simulink library "courseFollow_cl"  (R2018b)
settings: Solver=VariableStepAuto  StartTime=0.0  StopTime=10.0  RelTol=1e-3
undefined symbols (not defined in the file): a
libraries: $bdroot x6, schmehlTangentRotation_ul x2, dspindex x1, vectorNormalizer_ul x1, angleBtw2DVecs_ul x1, tangVecToPath x1
settings Model: Creator=James Reed  LastModifiedBy=James Reed

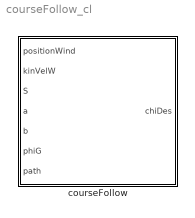
== system courseFollow_cl ==
  courseFollow : Subsystem

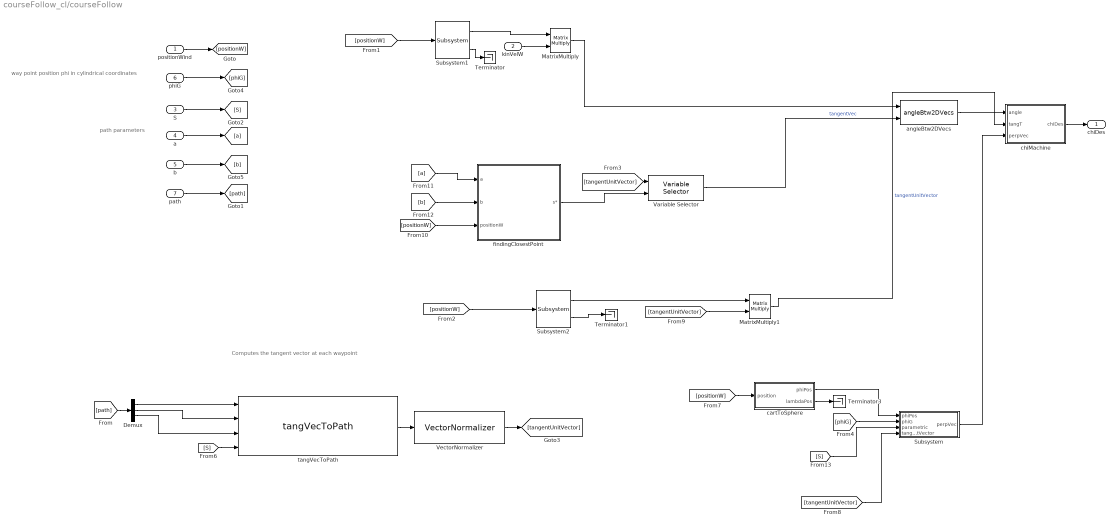
== system courseFollow_cl/courseFollow ==
  note: way point position phi in cylindrical coordinates
  note: path parameters
  note: Computes the tangent vector at each waypoint
  "positionWind " : Inport
  kinVelW : Inport  Port=2
  S : Inport  Port=3
  a : Inport  Port=4
  "b " : Inport  Port=5
  phiG : Inport  Port=6
  path : Inport  Port=7
  Demux : Demux  Outputs=3
  MatrixMultiply : Product  Multiplication=Matrix(*)
  MatrixMultiply1 : Product  Multiplication=Matrix(*)
  Subsystem : Subsystem
  Subsystem1 : schmehlTangentRotation_ul/Subsystem  SystemSampleTime=-1
  Subsystem2 : schmehlTangentRotation_ul/Subsystem  SystemSampleTime=-1
  Terminator : Terminator
  Terminator1 : Terminator
  Terminator3 : Terminator
  Variable Selector : dspindex/Variable Selector  NumInputs=1  rowsOrCols=Columns  IdxMode=Variable  Elements=[1 3]  ZerOneIdxMode=One-based  errmode=Clip Index  FillMode=on  FillValues=0
  "VectorNormalizer " : vectorNormalizer_ul/VectorNormalizer   SystemSampleTime=-1
  angleBtw2DVecs : angleBtw2DVecs_ul/angleBtw2DVecs  SystemSampleTime=-1
  cartToSphere : Subsystem
  chiMachine : Subsystem
  findingClosestPoint : Subsystem
  tangVecToPath : tangVecToPath/tangVecToPath  SystemSampleTime=-1
  "chiDes " : Outport
  wires:
  tangVecToPath/1 -> "VectorNormalizer "/1
  MatrixMultiply1/1 -> chiMachine/2(tangT)  "tangentUnitVector"
  Variable Selector/1 -> angleBtw2DVecs/2  "tangentVec"
  Subsystem1/2 -> Terminator/1
  kinVelW/1 -> MatrixMultiply/2
  Subsystem1/1 -> MatrixMultiply/1
  MatrixMultiply/1 -> angleBtw2DVecs/1
  Subsystem2/2 -> Terminator1/1
  "positionWind "/1 -> [positionW]
  [positionW] -> Subsystem1/1
  Subsystem2/1 -> MatrixMultiply1/1
  Demux/2 -> tangVecToPath/2
  Demux/3 -> tangVecToPath/3
  angleBtw2DVecs/1 -> chiMachine/1("angle ")
  chiMachine/1("chiDes ") -> "chiDes "/1
  cartToSphere/1(phiPos) -> Subsystem/1(phiPos)
  S/1 -> [S]
  [S] -> tangVecToPath/4
  [positionW] -> cartToSphere/1("position ")
  cartToSphere/2(lambdaPos) -> Terminator3/1
  "VectorNormalizer "/1 -> [tangentUnitVector]
  [tangentUnitVector] -> Subsystem/4("tangentUnitVector ")
  [tangentUnitVector] -> MatrixMultiply1/2
  [positionW] -> Subsystem2/1
  [positionW] -> findingClosestPoint/3(positionW)
  a/1 -> [a]
  "b "/1 -> [b]
  [a] -> findingClosestPoint/1(a)
  [b] -> findingClosestPoint/2(b)
  [S] -> Subsystem/3("parametric ")
  path/1 -> [path]
  [path] -> Demux/1
  Demux/1 -> tangVecToPath/1
  [tangentUnitVector] -> Variable Selector/1
  findingClosestPoint/1(s*) -> Variable Selector/2
  phiG/1 -> [phiG]
  Subsystem/1(perpVec) -> chiMachine/3("perpVec ")
  [phiG] -> Subsystem/2(phiG)

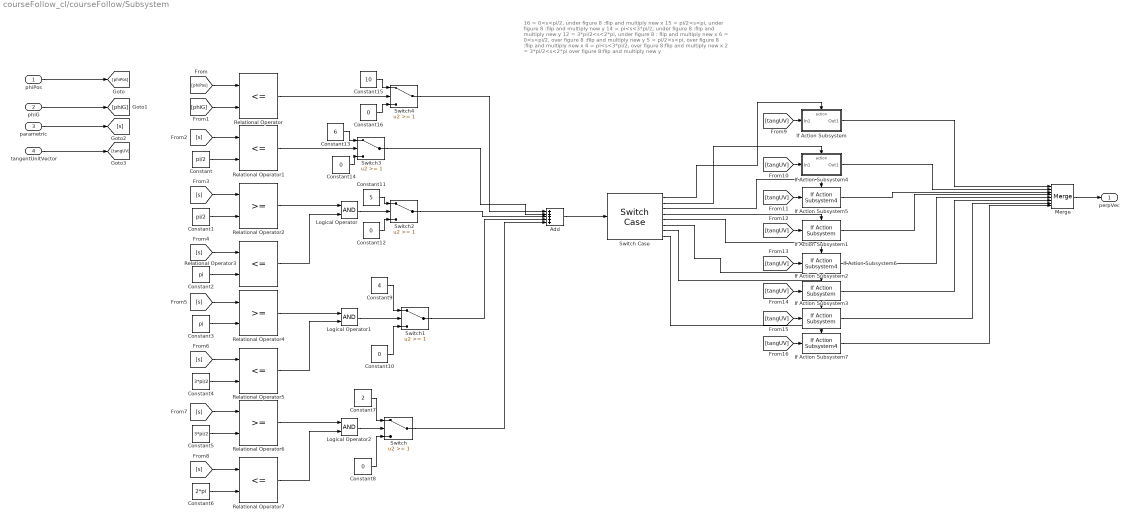
== system courseFollow_cl/courseFollow/Subsystem ==
  note: 16 = 0<s<pi/2, under figure 8 :flip and multiply new x
      | 15 = pi/2<s<pi, under figure 8  :flip and multiply new y
      | 14 = pi<s<3*pi/2, under figure 8 :flip and multiply new y
      | 12 = 3*pi/2<s<2*pi, under figure 8 : flip and multiply new x
      | 6 = 0<s<pi/2, over figure 8 :flip and multiply new y
      | 5 = pi/2<s<pi, over figure 8 :flip and multiply new x
      | 4 = pi<s<3*pi/2, over figure 8:flip and multiply new x
      | 2 = 3*pi/2<s<2*pi over figure 8:flip and multiply new y
  phiPos : Inport
  phiG : Inport  Port=2
  "parametric " : Inport  Port=3
  "tangentUnitVector " : Inport  Port=4
  Add : Sum  Inputs=+++++
  Constant : Constant  Value=pi/2
  Constant1 : Constant  Value=pi/2
  Constant{8,10,12,14,16} (5 alike) : Constant  Value=0
  Constant11 : Constant  Value=5
  Constant13 : Constant  Value=6
  Constant15 : Constant  Value=10
  Constant2 : Constant  Value=pi
  Constant3 : Constant  Value=pi
  Constant4 : Constant  Value=3*pi/2
  Constant5 : Constant  Value=3*pi/2
  Constant6 : Constant  Value=2*pi
  Constant7 : Constant  Value=2
  Constant9 : Constant  Value=4
  If Action Subsystem : Subsystem  TreatAsAtomicUnit=on
  If Action Subsystem1 : $bdroot/courseFollow/Subsystem/If Action Subsystem  SystemSampleTime=-1
  If Action Subsystem2 : $bdroot/courseFollow/Subsystem/If Action Subsystem  SystemSampleTime=-1
  If Action Subsystem3 : $bdroot/courseFollow/Subsystem/If Action Subsystem  SystemSampleTime=-1
  If Action Subsystem4 : Subsystem  TreatAsAtomicUnit=on
  If Action Subsystem5 : $bdroot/courseFollow/Subsystem/If Action Subsystem4  SystemSampleTime=-1
  If Action Subsystem6 : $bdroot/courseFollow/Subsystem/If Action Subsystem4  SystemSampleTime=-1
  If Action Subsystem7 : $bdroot/courseFollow/Subsystem/If Action Subsystem4  SystemSampleTime=-1
  Logical Operator : Logic  AllPortsSameDT=off  OutDataTypeStr=boolean
  Logical Operator1 : Logic  AllPortsSameDT=off  OutDataTypeStr=boolean
  Logical Operator2 : Logic  AllPortsSameDT=off  OutDataTypeStr=boolean
  Merge : Merge  Inputs=8
  Relational Operator{,1,3,5,7} (5 alike) : RelationalOperator  Operator=<=  OutDataTypeStr=boolean  RndMeth=Simplest
  Relational Operator2 : RelationalOperator  OutDataTypeStr=boolean  RndMeth=Simplest
  Relational Operator4 : RelationalOperator  OutDataTypeStr=boolean  RndMeth=Simplest
  Relational Operator6 : RelationalOperator  OutDataTypeStr=boolean  RndMeth=Simplest
  Switch{,1..4} (5 alike) : Switch  Threshold=1
  Switch Case : SwitchCase  CaseConditions={16,15,14,12,6,5,4,2}  ShowDefaultCase=off
  perpVec : Outport
  wires:
  phiPos/1 -> [phiPos]
  phiG/1 -> [phiG]
  Relational Operator/1 -> Switch4/2
  [phiPos] -> Relational Operator/1
  [phiG] -> Relational Operator/2
  "parametric "/1 -> [s]
  [s] -> Relational Operator1/1
  Constant/1 -> Relational Operator1/2
  [s] -> Relational Operator2/1
  Constant1/1 -> Relational Operator2/2
  Relational Operator2/1 -> Logical Operator/1
  [s] -> Relational Operator3/1
  Constant2/1 -> Relational Operator3/2
  Relational Operator3/1 -> Logical Operator/2
  Relational Operator4/1 -> Logical Operator1/1
  [s] -> Relational Operator4/1
  Constant4/1 -> Relational Operator5/2
  Constant3/1 -> Relational Operator4/2
  [s] -> Relational Operator5/1
  Relational Operator5/1 -> Logical Operator1/2
  Relational Operator6/1 -> Logical Operator2/1
  [s] -> Relational Operator6/1
  Constant6/1 -> Relational Operator7/2
  Constant5/1 -> Relational Operator6/2
  [s] -> Relational Operator7/1
  Relational Operator7/1 -> Logical Operator2/2
  Logical Operator2/1 -> Switch/2
  Constant7/1 -> Switch/1
  Constant8/1 -> Switch/3
  Logical Operator1/1 -> Switch1/2
  Constant9/1 -> Switch1/1
  Constant10/1 -> Switch1/3
  Logical Operator/1 -> Switch2/2
  Constant11/1 -> Switch2/1
  Constant12/1 -> Switch2/3
  Constant13/1 -> Switch3/1
  Constant14/1 -> Switch3/3
  Relational Operator1/1 -> Switch3/2
  Constant15/1 -> Switch4/1
  Constant16/1 -> Switch4/3
  Switch4/1 -> Add/1
  Switch3/1 -> Add/2
  Switch2/1 -> Add/3
  Switch1/1 -> Add/4
  Switch/1 -> Add/5
  Add/1 -> Switch Case/1
  Switch Case/1 -> If Action Subsystem/Action
  Switch Case/2 -> If Action Subsystem4/Action
  Switch Case/3 -> If Action Subsystem5/Action
  Switch Case/4 -> If Action Subsystem1/Action
  Switch Case/5 -> If Action Subsystem6/Action
  Switch Case/6 -> If Action Subsystem2/Action
  Switch Case/7 -> If Action Subsystem3/Action
  Switch Case/8 -> If Action Subsystem7/Action
  "tangentUnitVector "/1 -> [tangUV]
  [tangUV] -> If Action Subsystem/1(In1)
  [tangUV] -> If Action Subsystem4/1(In1)
  [tangUV] -> If Action Subsystem5/1
  [tangUV] -> If Action Subsystem1/1
  [tangUV] -> If Action Subsystem6/1
  [tangUV] -> If Action Subsystem2/1
  [tangUV] -> If Action Subsystem3/1
  [tangUV] -> If Action Subsystem7/1
  If Action Subsystem/1(Out1) -> Merge/1
  If Action Subsystem4/1(Out1) -> Merge/2
  If Action Subsystem5/1 -> Merge/3
  If Action Subsystem1/1 -> Merge/4
  If Action Subsystem6/1 -> Merge/5
  If Action Subsystem2/1 -> Merge/6
  If Action Subsystem3/1 -> Merge/7
  If Action Subsystem7/1 -> Merge/8
  Merge/1 -> perpVec/1

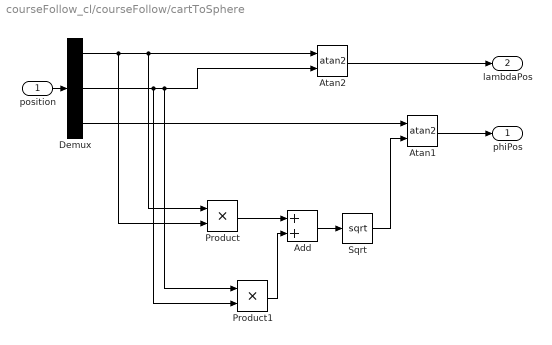
== system courseFollow_cl/courseFollow/cartToSphere ==
  "position " : Inport
  Add : Sum
  Atan1 : Trigonometry  Operator=atan2
  Atan2 : Trigonometry  Operator=atan2
  Demux : Demux  Outputs=3
  Product : Product
  Product1 : Product
  Sqrt : Sqrt  SaturateOnIntegerOverflow=on
  phiPos : Outport
  lambdaPos : Outport  Port=2
  wires:
  "position "/1 -> Demux/1
  Demux/1 -> Product/2, Product/1, Atan2/1
  Atan2/1 -> lambdaPos/1
  Demux/3 -> Atan1/1
  Atan1/1 -> phiPos/1
  Product/1 -> Add/1
  Add/1 -> Sqrt/1
  Demux/2 -> Product1/2, Product1/1, Atan2/2
  Product1/1 -> Add/2
  Sqrt/1 -> Atan1/2

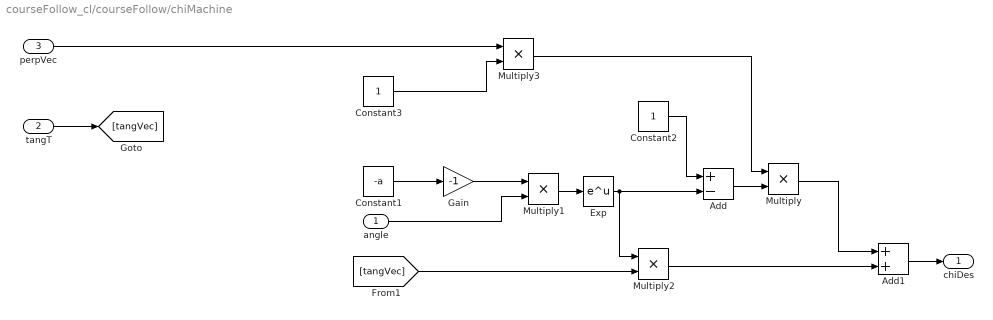
== system courseFollow_cl/courseFollow/chiMachine ==
  "angle " : Inport
  tangT : Inport  Port=2
  "perpVec " : Inport  Port=3
  Add : Sum  Inputs=+-
  Add1 : Sum
  Constant1 : Constant  Value=-a
  Constant2 : Constant
  Constant3 : Constant
  Exp : Math  SaturateOnIntegerOverflow=on
  Gain : Gain  Gain=-1
  Multiply{,1..3} (4 alike) : Product
  "chiDes " : Outport
  wires:
  tangT/1 -> [tangVec]
  Constant1/1 -> Gain/1
  Gain/1 -> Multiply1/1
  "angle "/1 -> Multiply1/2
  Multiply1/1 -> Exp/1
  Exp/1 -> Add/2, Multiply2/1
  Constant2/1 -> Add/1
  [tangVec] -> Multiply2/2
  Multiply3/1 -> Multiply/1
  Constant3/1 -> Multiply3/2
  Add/1 -> Multiply/2
  Multiply/1 -> Add1/1
  Multiply2/1 -> Add1/2
  Add1/1 -> "chiDes "/1
  "perpVec "/1 -> Multiply3/1

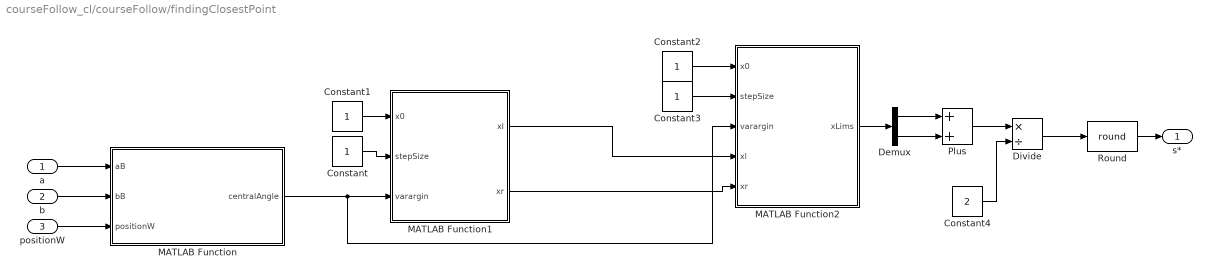
== system courseFollow_cl/courseFollow/findingClosestPoint ==
  a : Inport
  b : Inport  Port=2
  positionW : Inport  Port=3
  Constant{,1..3} (4 alike) : Constant
  Constant4 : Constant  Value=2
  Demux : Demux  Outputs=2
  Divide : Product  Inputs=*/
  MATLAB Function : MATLAB Function  TreatAsAtomicUnit=on
  MATLAB Function1 : MATLAB Function  TreatAsAtomicUnit=on
  MATLAB Function2 : MATLAB Function  TreatAsAtomicUnit=on
  Plus : Sum
  Round : Rounding  Operator=round
  s* : Outport
  wires:
  Constant2/1 -> MATLAB Function2/1(x0)
  Constant3/1 -> MATLAB Function2/2(stepSize)
  Constant1/1 -> MATLAB Function1/1(x0)
  Constant/1 -> MATLAB Function1/2(stepSize)
  MATLAB Function/1(centralAngle) -> MATLAB Function2/3(varargin), MATLAB Function1/3(varargin)
  MATLAB Function1/1(xl) -> MATLAB Function2/4(xl)
  MATLAB Function1/2(xr) -> MATLAB Function2/5(xr)
  MATLAB Function2/1(xLims) -> Demux/1
  Demux/2 -> Plus/2
  Demux/1 -> Plus/1
  Plus/1 -> Divide/1
  Constant4/1 -> Divide/2
  Divide/1 -> Round/1
  Round/1 -> s*/1
  a/1 -> MATLAB Function/1(aB)
  b/1 -> MATLAB Function/2(bB)
  positionW/1 -> MATLAB Function/3(positionW)

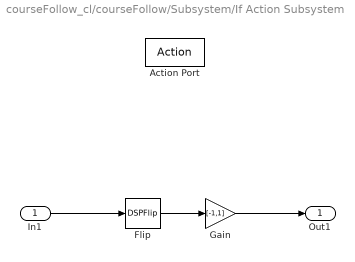
== system courseFollow_cl/courseFollow/Subsystem/If Action Subsystem ==
  In1 : Inport
  Action Port : ActionPort  ActionType=case
  Flip : DSPFlip
  Gain : Gain  Gain=[-1,1]
  Out1 : Outport
  wires:
  In1/1 -> Flip/1
  Flip/1 -> Gain/1
  Gain/1 -> Out1/1

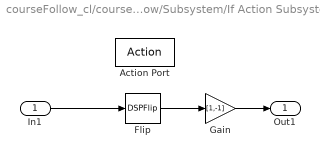
== system courseFollow_cl/courseFollow/Subsystem/If Action Subsystem4 ==
  In1 : Inport
  Action Port : ActionPort  ActionType=case
  Flip : DSPFlip
  Gain : Gain  Gain=[1,-1]
  Out1 : Outport
  wires:
  Flip/1 -> Gain/1
  In1/1 -> Flip/1
  Gain/1 -> Out1/1

== matlab function courseFollow_cl/courseFollow/findingClosestPoint/MATLAB Function ==
  data: aB input; centralAngle output; bB input; positionW input
function centralAngle  = fcn(aB,bB,positionW)

lambda_g = (aB.*sin(s))./(1 + ((aB/bB)^2).*(cos(s).^2)); %path longitude
phi_g  = (10*pi/180)+(((aB/bB)^2).*sin(s).*cos(s))./(1 + ((aB/bB)^2).*(cos(s).^2)); %path latitude

path = [ cos(lambda_g).*cos(phi_g);
         sin(lambda_g).*cos(phi_g);
         sin(phi_g);]; 
      pathFunction = @(s) path ;
     centralAngle = @(s)2*asin(.5*(norm(pathFunction(s)-currentPosition)));

== matlab function courseFollow_cl/courseFollow/findingClosestPoint/MATLAB Function1 ==
  data: x0 input; xl output; stepSize input; varargin input; xr output
function [xl,xr] = bound(x0, stepSize,varargin)

p = inputParser;

% Number of iterations before stopping attempt to tune step size
addOptional(p,'StepTimeout',1000,@(x) isnumeric(x) && isscalar(x))
% How much to increase the step size at every iteration
addOptional(p,'StepSizeMultiplier',2,@(x) isnumeric(x) && isscalar(x)  && x>=1)
% Number of iterations before quitting bounding phase
addOptional(p,'BoundingTimeout',1000,@(x) isnumeric(x) && isscalar(x))
% Handle of the function that you want to minimize
addOptional(p,'FunctionHandle',@objF,@(x) isa(x,'function_handle'))
% Initial point/guess
addRequired(p,'x0',@(x) isnumeric(x) && isvector(x))
% Step size
addRequired(p,'StepSize',@(x) isnumeric(x) && isscalar(x) && x>0)

parse(p,x0,stepSize,varargin{:})

fHandle  = p.Results.FunctionHandle;
stepSize = p.Results.StepSize;
x0       = p.Results.x0;

for tryCount = 1:p.Results.StepTimeout
    if fHandle(x0-stepSize) >= fHandle(x0) &&...
            fHandle(x0) >= fHandle(x0+stepSize)
        sign = +1;
        break
    elseif  fHandle(x0-stepSize) <= fHandle(x0) &&...
            fHandle(x0) <= fHandle(x0+stepSize)
        sign = -1;
        break
    end
    stepSize = stepSize/2^tryCount;
end

xCurrent = x0;
for ii = 0:p.Results.BoundingTimeout-1
    xRight = xCurrent + sign*stepSize*p.Results.StepSizeMultiplier^ii;
    if fHandle(xRight)>fHandle(xCurrent)
        break
    end
    xLeft = xCurrent;
    xCurrent = xRight;
end

if sign == -1
   xTemp  = sort([xLeft xRight]) ;
   xl  = xTemp(1);
   xr = xTemp(2);
end

end

== matlab function courseFollow_cl/courseFollow/findingClosestPoint/MATLAB Function2 ==
  data: x0 input; xLims output; stepSize input; varargin input; xl input; xr input
function xLims = goldenSection(x0,stepSize,varargin,xl,xr)
% Function to implement golden section to minimize a scalar function
%
% Required Inputs
% x0       - initial guess
% stepSize - initial step size (step size may be reduced if this is too
% big)
%
% Optional Inputs
% DisplayOutput -  true/false prints output to command window
% MaxIterations - Maximum number of iterations before quitting, default =
% 1000
% FunctionConvergence - convergence criteria for function value, set to
% zero to disable, default = 0.01
% InputConvergence - convergence criteria for function input, set to zero
% to disable, default = 0.01
% StepTimeout - Max number of iterations for bounding phase step size
% reduction, default = 1000
% BoundingTimeout - Max number of iterations for bounding phase, default =
% 1000
 

% Input parsing
p = inputParser;
addRequired(p,'x0',@(x) isnumeric(x) && isscalar(x))
addRequired(p,'StepSize',@(x) isnumeric(x) && isscalar(x) && x>0)
addOptional(p,'DisplayOutput',false,@(x) islogical(x))
addOptional(p,'MaxIterations',1000,@(x) isnumeric(x) && isscalar(x) && x>0)
addOptional(p,'FunctionConvergence',0.00001,@(x) isnumeric(x) && isscalar(x) && x>=0)
addOptional(p,'InputConvergence',0.0001,@(x) isnumeric(x) && isscalar(x) && x>=0)
addOptional(p,'StepTimeout',1000,@(x) isnumeric(x) && isscalar(x))
addOptional(p,'StepSizeMultiplier',2,@(x) isnumeric(x) && isscalar(x)  && x>=1)
addOptional(p,'BoundingTimeout',1000,@(x) isnumeric(x) && isscalar(x))
addOptional(p,'FunctionHandle',@objF,@(x) isa(x,'function_handle'))
parse(p,x0,stepSize,varargin{:})

% Rename some variables to clean up code later on
fHandle  = p.Results.FunctionHandle;
stepSize = p.Results.StepSize;
x0       = p.Results.x0;

% Bounding Phase
[xl,xr] = bound(x0,stepSize,'FunctionHandle',p.Results.FunctionHandle,...
    'StepTimeout',p.Results.StepTimeout,...
    'StepSizeMultiplier',p.Results.StepSizeMultiplier,...
    'BoundingTimeout',p.Results.BoundingTimeout,...
    'FunctionHandle',p.Results.FunctionHandle);

% Begin golden section
tau = 1 - 0.38197;
initialRange = abs(xr-xl);
fl = fHandle(xl);
fr = fHandle(xr);
% Print column headers to command window for output
if p.Results.DisplayOutput
    headings = {'xl','Fl','x1','F1','x2','F2','xr','Fr','xOpt','FOpt'};
    headingString = [' '];
    for ii = 1:length(headings)
        headingString = [headingString pad(headings{ii},11)];
    end
    fprintf(['\n' headingString '\n'])
end

for ii = 1:p.Results.MaxIterations
    xTwo = (1-tau)*xl+tau*xr;
    xOne = tau*xl+(1-tau)*xr;
    fOne = fHandle(xOne);
    fTwo = fHandle(xTwo);
    fMin = min([fl fr fOne fTwo]);
    fMax = max([fl fr fOne fTwo]);
    xMin = min([xl xr xOne xTwo]);
    xMax = max([xl xr xOne xTwo]);
    if abs((fMax-fMin)/fMin)<= p.Results.FunctionConvergence || ...
            abs((xMax - xMin)/initialRange) <= p.Results.InputConvergence
        if p.Results.DisplayOutput
            fprintf('\nSolution converged.  Stopping program.\n')
        end
        break
    end
    if fOne>fTwo
        xl = xOne;
        f1 = fOne;
    else
        xr = xTwo;
        fr = fTwo;
    end
end

% xTest = linspace(-1,1,1000);
% for ii = 1:length(xTest)
%     y(ii) = fHandle(xTest(ii));
% end
% plot(xTest,y)

xLims = [xl xr];
end
